simulink model "resistor_inductor_circut"  (R2024b)
settings: Solver=FixedStepAuto  StartTime=0.0  StopTime=10  FixedStep=0.0001  RelTol=1e-3
settings Model: Creator=castl  LastModifiedBy=castl

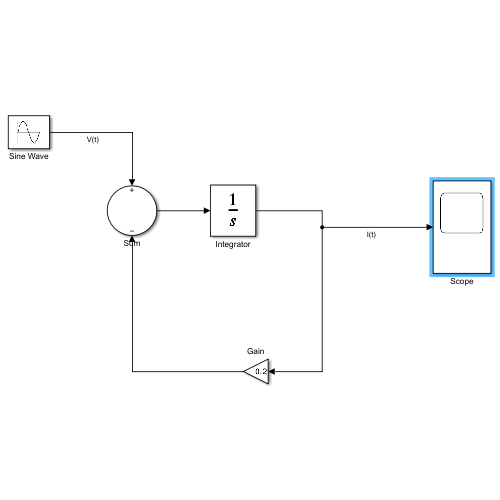
[thumbnail: Simulink's stored preview of the top-level diagram]
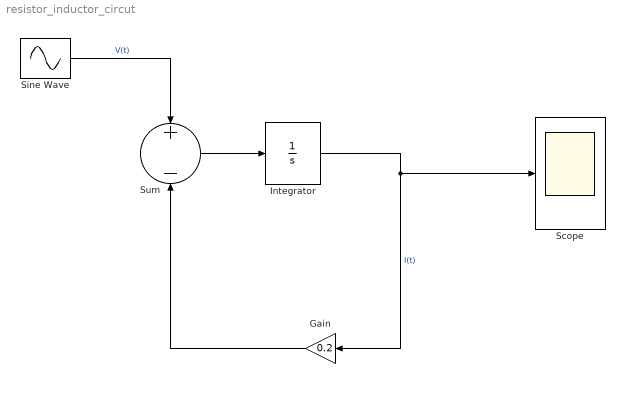
== system resistor_inductor_circut ==
  Gain : Gain  Gain=0.2
  Integrator : Integrator
  Scope : Scope
  Sine Wave : Sin  Amplitude=10  Phase=pi/4  SampleTime=0
  Sum : Sum  Inputs=+-
  wires:
  Sine Wave/1 -> Sum/1  "V(t)"
  Sum/1 -> Integrator/1
  Integrator/1 -> Scope/1, Gain/1  "I(t)"
  Gain/1 -> Sum/2
